simulink model "Square_Wave_Injection"  (R2023b)
settings: Solver=VariableStepAuto  StartTime=0.0  StopTime=3  RelTol=1e-3
undefined symbols (not defined in the file or in its folder): DiscIntNeverNeededParam
libraries: spsDCVoltageSourceLib x1, spsPermanentMagnetSynchronousMachineLib x1, simulink x1, spsUniversalBridgeLib x1, sps_lib x1
settings Model: Creator=yfp  LastModifiedBy=13571
settings SolverCC: AlgebraicLoopSolver=TrustRegion
settings OptimizationCC: ReuseModelBlockBuffer=off
settings DebuggingCC: UnconnectedInputMsg=warning  UnconnectedOutputMsg=warning  UnconnectedLineMsg=warning  ArithmeticOperatorsInVariantConditions=warning
settings ModelReferenceCC: EnableRefExpFcnMdlSchedulingChecks=on
settings SFSimCC: CustomCodeUndefinedFunction=UseInterfaceOnly

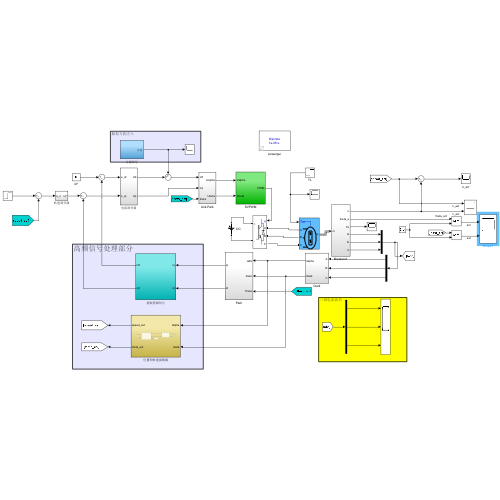
[thumbnail: Simulink's stored preview of the top-level diagram]
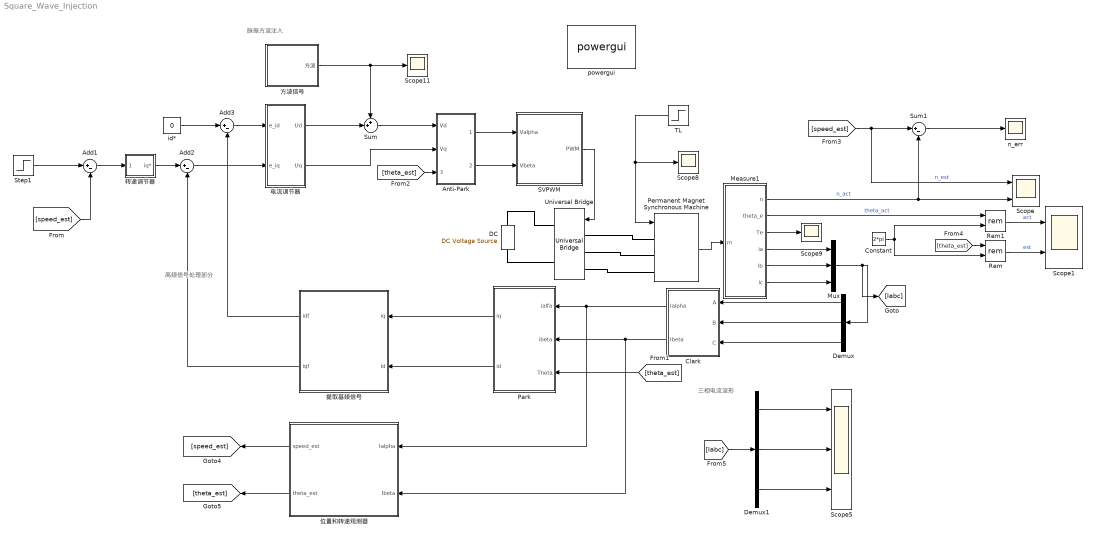
== system Square_Wave_Injection ==
  note: 三相电流波形
  note: 脉振方波注入
  note: 高频信号处理部分
  Add1 : Sum  Inputs=|+-
  Add2 : Sum  Inputs=|+-
  Add3 : Sum  Inputs=|+-
  Anti-Park : Subsystem
  Clark : Subsystem
  Constant : Constant  Value=2*pi
  "DC " : spsDCVoltageSourceLib/DC Voltage Source  Amplitude=300  Measurements=None
  Demux : Demux  Outputs=3
  Demux1 : Demux  Outputs=3
  Measure1 : Subsystem
  Mux : Mux  Inputs=3
  "Park " : Subsystem
  Permanent Magnet Synchronous Machine : spsPermanentMagnetSynchronousMachineLib/Permanent Magnet Synchronous Machine  NbPhases=3  FluxDistribution=Sinusoidal  RotorType=Salient-pole  MechanicalLoad=Torque Tm  PresetModel=No  ShowDetailedParameters=on  MeasurementBus=off  Resistance=0.045  Inductance=8.5e-3  dqInductances=[130e-6,235e-6]  La=0.000835  MachineConstant=Flux linkage established by magnets (V.s)  Flux=0.048517  VoltageCst=35.2  TorqueCst=0.2911  Flat=120  Mechanical=[0.0034 0.005 4 0]  PolePairs=4  InitialConditions=[0,0, 0,0]  InitialConditions5ph=[0 0 0 0 0 0]  RefAngle=Aligned with phase A axis (original Park)  IterativeDiscreteModel=Trapezoidal non iterative  TsBlock=-1  TsPowergui=0
  Rem : Math  Operator=rem  SignedPower=on
  Rem1 : Math  Operator=rem  SignedPower=on
  SVPWM : Subsystem
  Scope : Scope  NumInputPorts=2
  Scope1 : Scope  NumInputPorts=2
  Scope11 : Scope
  Scope5 : Scope  NumInputPorts=3
  Scope8 : Scope
  Scope9 : Scope
  Step1 : Step  Time=0  After=200  SampleTime=0
  Sum : Sum  Inputs=++|
  Sum1 : Sum  Inputs=|+-
  TL : Step  Time=0.5  SampleTime=0
  Universal Bridge : spsUniversalBridgeLib/Universal Bridge  Arms=3  SnubberResistance=1e5  SnubberCapacitance=inf  Device=IGBT / Diodes  Ron=1e-3  Lon=0  ForwardVoltages="[  0  0  ]"  ForwardVoltage=0  GTOparameters=[ 10e-6 , 20e-6 ]  IGBTparameters=[ 1e-6 , 2e-6 ]  Measurements=None  Measurements_2=None  converterType=Rectifier
  id* : Constant  Value=0
  n_err : Scope
  powergui : sps_lib/powergui  Priority=1  SimulationMode=Discrete  SampleTime=1e-6  frequency=60  Iterations=50  frequencyindice=0  Pbase=100e6  ErrMax=1e-4  UnitsV=kV  UnitsW=MW  buscounter=0  FunctionMessages=off  echomessages=off  EnableUseOfTLC=off  CurrentSourceSwitches=off  DisableSnubberDevices=off  DisableRonSwitches=off  DisableVfSwitches=off  DisplayEquations=off  AutomaticDiscreteSolvers=off  SolverType=Tustin/Backward Euler (TBE)  Interpol=off  ExternalGateDelay=off  methode=off  Ts=100  x0status=blocks  SPID=on  SwTol=0  HookPort=off  NonlinearTolerance=1e-4  nMaxIteration=100  ContinueOnMaxIteration=off  RestoreLinks=warning  ResistiveCurrentMeasurement=off  Frange=[0:2:500]  Ylog=off  Xlog=on  ShowGrid=off  save=off  variable=ZData  structure=iq  ZoomFFT=off  StartTime=0.1  cycles=100  DisplayStyle=2  fundamental=1000  FreqAxis=off  MaxFrequency=10000  frequencyindicesteady=1  RmsSteady=1  display=off
  位置和转速观测器 : Subsystem
  提取基频信号 : Subsystem
  方波信号 : Subsystem
  电流调节器 : Subsystem
  转速调节器 : Subsystem
  wires:
  Measure1/2(theta_e) -> Rem1/1  "theta_act"
  Sum/1 -> Anti-Park/1(Vd)
  Demux/2 -> Clark/2(B)
  Measure1/1(n) -> Sum1/2, Scope/2  "n_act"
  电流调节器/2(Uq) -> Anti-Park/2(Vq)
  电流调节器/1(Ud) -> Sum/2
  [speed_est] -> Scope/1, Sum1/1  "n_est"
  Step1/1 -> Add1/1
  Measure1/5(ib) -> Mux/2
  Sum1/1 -> n_err/1
  位置和转速观测器/2(theta_est) -> [theta_est]
  Add1/1 -> 转速调节器/1(e_n)
  Clark/2(Ibeta) -> 位置和转速观测器/2(Ibeta), "Park "/2(ibeta)
  位置和转速观测器/1(speed_est) -> [speed_est]
  Constant/1 -> Rem1/2, Rem/2
  Add2/1 -> 电流调节器/2(e_iq)
  "Park "/2(id) -> 提取基频信号/2(id)
  提取基频信号/1(idf) -> Add3/2
  Permanent Magnet Synchronous Machine/1 -> Measure1/1(m)
  Mux/1 -> [Iabc], Demux/1
  Demux/3 -> Clark/3(C)
  Measure1/3(Te) -> Scope9/1
  [theta_est] -> Rem/1
  TL/1 -> Scope8/1, Permanent Magnet Synchronous Machine/1
  Measure1/6(ic) -> Mux/3
  方波信号/1(方波) -> Scope11/1, Sum/1
  "Park "/1(iq) -> 提取基频信号/1(iq)
  Anti-Park/2(Ubeta) -> SVPWM/2(Vbeta)
  Measure1/4(ia) -> Mux/1
  Rem/1 -> Scope1/2  "est"
  Anti-Park/1(Ualpha) -> SVPWM/1(Valpha)
  Demux/1 -> Clark/1(A)
  Add3/1 -> 电流调节器/1(e_id)
  id*/1 -> Add3/1
  Rem1/1 -> Scope1/1  "act"
  提取基频信号/2(iqf) -> Add2/2
  Clark/1(Ialpha) -> 位置和转速观测器/1(Ialpha), "Park "/1(ialfa)
  [speed_est] -> Add1/2
  [theta_est] -> Anti-Park/3(theta)
  [theta_est] -> "Park "/3(Theta)
  SVPWM/1(PWM) -> Universal Bridge/1
  转速调节器/1(iq*) -> Add2/1
  [Iabc] -> Demux1/1
  Demux1/1 -> Scope5/1
  Demux1/2 -> Scope5/2
  Demux1/3 -> Scope5/3
  connections:
  Permanent Magnet Synchronous Machine/LConn1 -- Universal Bridge/LConn1
  Permanent Magnet Synchronous Machine/LConn3 -- Universal Bridge/LConn3
  "DC "/LConn1 -- Universal Bridge/RConn2
  Universal Bridge/RConn1 -- "DC "/RConn1
  Permanent Magnet Synchronous Machine/LConn2 -- Universal Bridge/LConn2

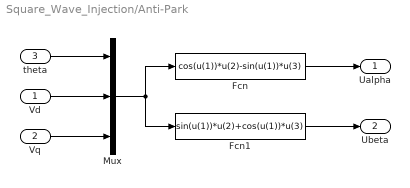
== system Square_Wave_Injection/Anti-Park ==
  Vd : Inport
  Vq : Inport  Port=2
  theta : Inport  Port=3
  Fcn : Fcn  Expr=cos(u(1))*u(2)-sin(u(1))*u(3)
  Fcn1 : Fcn  Expr=sin(u(1))*u(2)+cos(u(1))*u(3)
  Mux : Mux  Inputs=3
  Ualpha : Outport  VectorParamsAs1DForOutWhenUnconnected=off
  Ubeta : Outport  Port=2  VectorParamsAs1DForOutWhenUnconnected=off
  wires:
  Vd/1 -> Mux/2
  Vq/1 -> Mux/3
  Mux/1 -> Fcn/1, Fcn1/1
  Fcn1/1 -> Ubeta/1
  Fcn/1 -> Ualpha/1
  theta/1 -> Mux/1

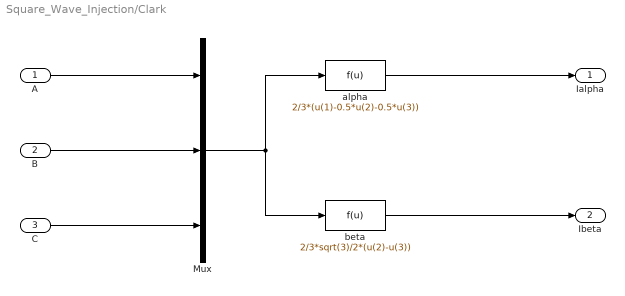
== system Square_Wave_Injection/Clark ==
  A : Inport
  B : Inport  Port=2
  C : Inport  Port=3
  Mux : Mux  Inputs=3
  alpha : Fcn  Expr=2/3*(u(1)-0.5*u(2)-0.5*u(3))
  beta : Fcn  Expr=2/3*sqrt(3)/2*(u(2)-u(3))
  Ialpha : Outport  VectorParamsAs1DForOutWhenUnconnected=off
  Ibeta : Outport  Port=2  VectorParamsAs1DForOutWhenUnconnected=off
  wires:
  Mux/1 -> beta/1, alpha/1
  alpha/1 -> Ialpha/1
  beta/1 -> Ibeta/1
  C/1 -> Mux/3
  A/1 -> Mux/1
  B/1 -> Mux/2

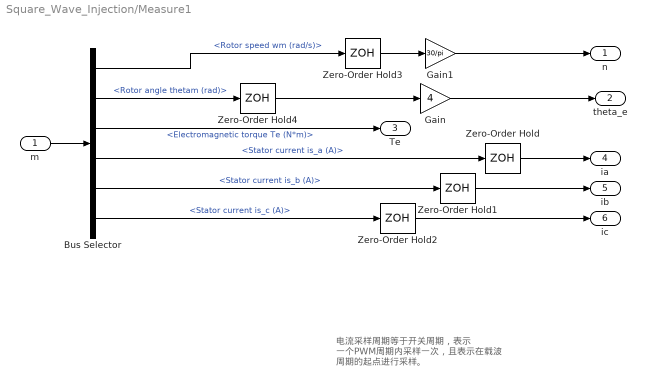
== system Square_Wave_Injection/Measure1 ==
  note: 电流采样周期等于开关周期，表示
      | 一个PWM周期内采样一次，且表示在载波
      | 周期的起点进行采样。
  m : Inport
  Bus Selector : BusSelector  OutputSignals=Rotor speed wm (rad/s),Rotor angle thetam (rad),Electromagnetic torque Te (N*m),Stator current is_a (A),Stator current is_b (A),Stator current is_c (A)
  Gain : Gain  Gain=4
  Gain1 : Gain  Gain=30/pi
  Zero-Order Hold{,1..4} (5 alike) : ZeroOrderHold  SampleTime=1e-4
  n : Outport  VectorParamsAs1DForOutWhenUnconnected=off
  theta_e : Outport  Port=2  VectorParamsAs1DForOutWhenUnconnected=off
  Te : Outport  Port=3  VectorParamsAs1DForOutWhenUnconnected=off
  ia : Outport  Port=4  VectorParamsAs1DForOutWhenUnconnected=off
  ib : Outport  Port=5  VectorParamsAs1DForOutWhenUnconnected=off
  ic : Outport  Port=6  VectorParamsAs1DForOutWhenUnconnected=off
  wires:
  m/1 -> Bus Selector/1
  Bus Selector/3 -> Te/1  "<Electromagnetic torque Te (N*m)>"
  Bus Selector/1 -> Zero-Order Hold3/1  "<Rotor speed wm (rad/s)>"
  Bus Selector/2 -> Zero-Order Hold4/1  "<Rotor angle thetam (rad)>"
  Bus Selector/4 -> Zero-Order Hold/1  "<Stator current is_a (A)>"
  Bus Selector/5 -> Zero-Order Hold1/1  "<Stator current is_b (A)>"
  Bus Selector/6 -> Zero-Order Hold2/1  "<Stator current is_c (A)>"
  Zero-Order Hold3/1 -> Gain1/1
  Zero-Order Hold4/1 -> Gain/1
  Zero-Order Hold/1 -> ia/1
  Zero-Order Hold1/1 -> ib/1
  Zero-Order Hold2/1 -> ic/1
  Gain/1 -> theta_e/1
  Gain1/1 -> n/1

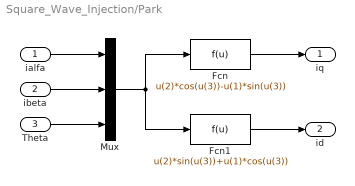
== system Square_Wave_Injection/Park  ==
  ialfa : Inport
  ibeta : Inport  Port=2
  Theta : Inport  Port=3
  Fcn : Fcn  Expr=u(2)*cos(u(3))-u(1)*sin(u(3))
  Fcn1 : Fcn  Expr=u(2)*sin(u(3))+u(1)*cos(u(3))
  Mux : Mux  Inputs=3
  iq : Outport  VectorParamsAs1DForOutWhenUnconnected=off
  id : Outport  Port=2  VectorParamsAs1DForOutWhenUnconnected=off
  wires:
  Theta/1 -> Mux/3
  Fcn1/1 -> id/1
  Fcn/1 -> iq/1
  Mux/1 -> Fcn/1, Fcn1/1
  ibeta/1 -> Mux/2
  ialfa/1 -> Mux/1

== system Square_Wave_Injection/SVPWM ==
  Valpha : Inport
  Vbeta : Inport  Port=2
  CMPR : Scope
  Embedded MATLAB Function : MATLAB Function  TreatAsAtomicUnit=on
  Mux6 : Mux  Inputs=3
  Udc : Constant  Value=135
  pwm generator : Subsystem
  PWM : Outport  VectorParamsAs1DForOutWhenUnconnected=off
  wires:
  Embedded MATLAB Function/1(ta) -> Mux6/1, pwm generator/1(Ta)
  Embedded MATLAB Function/2(tb) -> Mux6/2, pwm generator/2(Tb)
  Embedded MATLAB Function/3(tc) -> Mux6/3, pwm generator/3(Tc)
  Mux6/1 -> CMPR/1
  pwm generator/1(pwm) -> PWM/1
  Valpha/1 -> Embedded MATLAB Function/1(Vsalpha)
  Vbeta/1 -> Embedded MATLAB Function/2(Vsbeta)
  Udc/1 -> Embedded MATLAB Function/3(Udc)

== system Square_Wave_Injection/位置和转速观测器 ==
  Ialpha : Inport
  Ibeta : Inport  Port=2
  两相静止坐标系提取高频信号 : Subsystem
  位置估算2 : Subsystem
  speed_est : Outport
  theta_est : Outport  Port=2
  wires:
  Ialpha/1 -> 两相静止坐标系提取高频信号/1(i_alpha)
  Ibeta/1 -> 两相静止坐标系提取高频信号/2(i_beta)
  两相静止坐标系提取高频信号/1(i_alpha_h) -> 位置估算2/1(Ialpha_h)
  两相静止坐标系提取高频信号/2(i_beta_h) -> 位置估算2/2(Ibeta_h)
  [Udh] -> 位置估算2/3(Udh)
  位置估算2/1(Speed_Est) -> speed_est/1
  位置估算2/2(theta_e^) -> theta_est/1

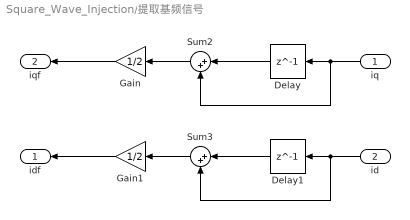
== system Square_Wave_Injection/提取基频信号 ==
  iq : Inport
  id : Inport  Port=2
  Delay : Delay  DelayLength=1  SampleTime=1e-4
  Delay1 : Delay  DelayLength=1  SampleTime=1e-4
  Gain : Gain  Gain=1/2
  Gain1 : Gain  Gain=1/2
  Sum2 : Sum  Inputs=|++
  Sum3 : Sum  Inputs=|++
  idf : Outport  VectorParamsAs1DForOutWhenUnconnected=off
  iqf : Outport  Port=2  VectorParamsAs1DForOutWhenUnconnected=off
  wires:
  Delay/1 -> Sum2/1
  Delay1/1 -> Sum3/1
  Sum3/1 -> Gain1/1
  id/1 -> Delay1/1, Sum3/2
  Gain1/1 -> idf/1
  Gain/1 -> iqf/1
  Sum2/1 -> Gain/1
  iq/1 -> Delay/1, Sum2/2

== system Square_Wave_Injection/方波信号 ==
  Constant : Constant  Value=20
  Pulse Generator : DiscretePulseGenerator  PulseType=Time based  Amplitude=40  Period=2e-4  PulseWidth=50
  Subtract : Sum  Inputs=+-
  方波 : Outport  VectorParamsAs1DForOutWhenUnconnected=off
  tag scope: Udh=global
  wires:
  Pulse Generator/1 -> Subtract/1
  Constant/1 -> Subtract/2
  Subtract/1 -> [Udh], 方波/1

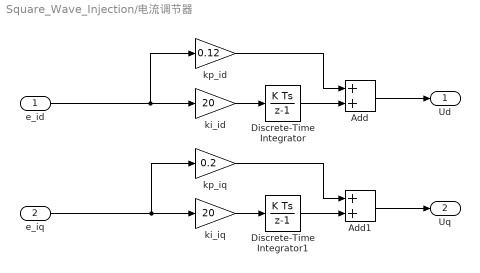
== system Square_Wave_Injection/电流调节器 ==
  e_id : Inport
  e_iq : Inport  Port=2
  Add : Sum
  Add1 : Sum
  Discrete-Time Integrator : DiscreteIntegrator  SampleTime=1e-4  LimitOutput=on  UpperSaturationLimit=135/1.732  LowerSaturationLimit=-135/1.732  ICPrevOutput=DiscIntNeverNeededParam  ICPrevScaledInput=DiscIntNeverNeededParam
  Discrete-Time Integrator1 : DiscreteIntegrator  SampleTime=1e-4  LimitOutput=on  UpperSaturationLimit=135/1.732  LowerSaturationLimit=-135/1.732  ICPrevOutput=DiscIntNeverNeededParam  ICPrevScaledInput=DiscIntNeverNeededParam
  ki_id : Gain  Gain=20
  ki_iq : Gain  Gain=20
  kp_id : Gain  Gain=0.12
  kp_iq : Gain  Gain=0.2
  Ud : Outport  VectorParamsAs1DForOutWhenUnconnected=off
  Uq : Outport  Port=2  VectorParamsAs1DForOutWhenUnconnected=off
  wires:
  ki_id/1 -> Discrete-Time Integrator/1
  Discrete-Time Integrator/1 -> Add/2
  kp_id/1 -> Add/1
  ki_iq/1 -> Discrete-Time Integrator1/1
  Discrete-Time Integrator1/1 -> Add1/2
  kp_iq/1 -> Add1/1
  Add/1 -> Ud/1
  Add1/1 -> Uq/1
  e_id/1 -> kp_id/1, ki_id/1
  e_iq/1 -> kp_iq/1, ki_iq/1

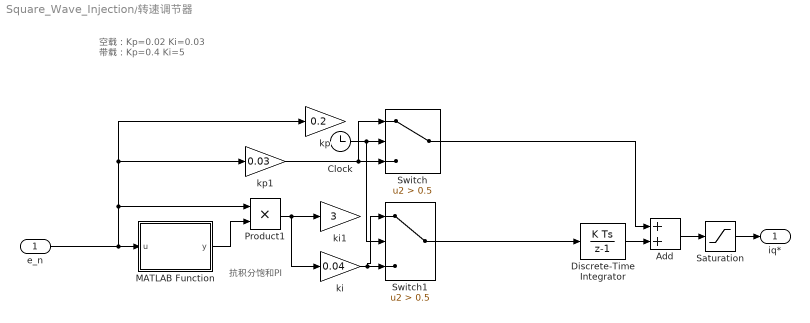
== system Square_Wave_Injection/转速调节器 ==
  note: 空载：Kp=0.02 Ki=0.03
      | 带载：Kp=0.4 Ki=5
  note: 抗积分饱和PI
  e_n : Inport
  Add : Sum
  Clock : Clock
  Discrete-Time Integrator : DiscreteIntegrator  SampleTime=1e-4  LimitOutput=on  UpperSaturationLimit=50  LowerSaturationLimit=-50  ICPrevOutput=DiscIntNeverNeededParam  ICPrevScaledInput=DiscIntNeverNeededParam
  MATLAB Function : MATLAB Function  TreatAsAtomicUnit=on
  Product1 : Product
  Saturation : Saturate  UpperLimit=50  LowerLimit=-50
  Switch : Switch  Criteria=u2 > Threshold  Threshold=0.5  SaturateOnIntegerOverflow=off  InputSameDT=off
  Switch1 : Switch  Criteria=u2 > Threshold  Threshold=0.5  SaturateOnIntegerOverflow=off  InputSameDT=off
  ki : Gain  Gain=0.04
  ki1 : Gain  Gain=3
  kp : Gain  Gain=0.2
  kp1 : Gain  Gain=0.03
  iq* : Outport  VectorParamsAs1DForOutWhenUnconnected=off
  wires:
  Discrete-Time Integrator/1 -> Add/2
  Add/1 -> Saturation/1
  MATLAB Function/1(y) -> Product1/2
  Saturation/1 -> iq*/1
  e_n/1 -> kp/1, kp1/1, Product1/1, MATLAB Function/1(u)
  Clock/1 -> Switch1/2, Switch/2
  Product1/1 -> ki/1, ki1/1
  Switch/1 -> Add/1
  Switch1/1 -> Discrete-Time Integrator/1
  ki/1 -> Switch1/1, Switch1/3
  kp1/1 -> Switch/1, Switch/3

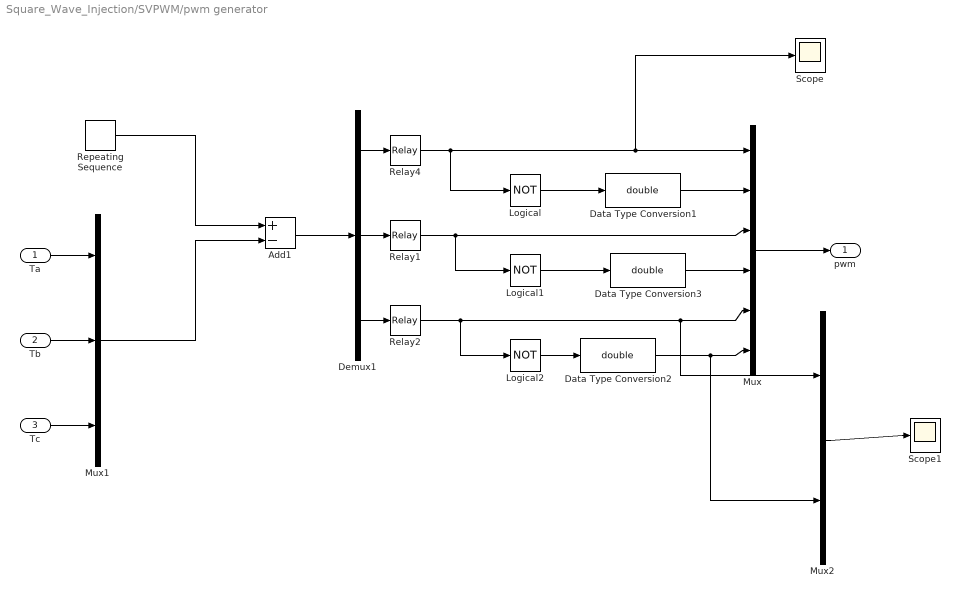
== system Square_Wave_Injection/SVPWM/pwm generator ==
  Ta : Inport
  Tb : Inport  Port=2
  Tc : Inport  Port=3
  Add1 : Sum  Inputs=+-
  Data Type Conversion1 : DataTypeConversion  OutDataTypeStr=double  SaturateOnIntegerOverflow=off  RndMeth=Floor
  Data Type Conversion2 : DataTypeConversion  OutDataTypeStr=double  SaturateOnIntegerOverflow=off  RndMeth=Floor
  Data Type Conversion3 : DataTypeConversion  OutDataTypeStr=double  SaturateOnIntegerOverflow=off  RndMeth=Floor
  Demux1 : Demux  Outputs=3
  "Logical " : Logic  Operator=NOT  AllPortsSameDT=off  OutDataTypeStr=boolean
  Logical1 : Logic  Operator=NOT  AllPortsSameDT=off  OutDataTypeStr=boolean
  Logical2 : Logic  Operator=NOT  AllPortsSameDT=off  OutDataTypeStr=boolean
  Mux : Mux  Inputs=6
  Mux1 : Mux  Inputs=3
  Mux2 : Mux  Inputs=2
  Relay1 : Relay  OnSwitchValue=0.00001  OffSwitchValue=-0.00001  OutDataTypeStr=Inherit: Inherit via back propagation
  Relay2 : Relay  OnSwitchValue=0.00001  OffSwitchValue=-0.00001  OutDataTypeStr=Inherit: Inherit via back propagation
  Relay4 : Relay  OnSwitchValue=0.00001  OffSwitchValue=-0.00001  OutDataTypeStr=Inherit: Inherit via back propagation
  Repeating Sequence : simulink/Sources/Repeating Sequence  rep_seq_t=[0 0.00005 0.0001]  rep_seq_y=[0 1 0]
  Scope : Scope
  Scope1 : Scope
  pwm : Outport  VectorParamsAs1DForOutWhenUnconnected=off
  wires:
  Repeating Sequence/1 -> Add1/1
  Demux1/1 -> Relay4/1
  Demux1/2 -> Relay1/1
  Demux1/3 -> Relay2/1
  Mux/1 -> pwm/1
  Add1/1 -> Demux1/1
  "Logical "/1 -> Data Type Conversion1/1
  Data Type Conversion1/1 -> Mux/2
  Logical1/1 -> Data Type Conversion3/1
  Data Type Conversion3/1 -> Mux/4
  Logical2/1 -> Data Type Conversion2/1
  Data Type Conversion2/1 -> Mux/6, Mux2/2
  Relay4/1 -> "Logical "/1, Mux/1, Scope/1
  Relay1/1 -> Logical1/1, Mux/3
  Relay2/1 -> Logical2/1, Mux/5, Mux2/1
  Ta/1 -> Mux1/1
  Tb/1 -> Mux1/2
  Tc/1 -> Mux1/3
  Mux1/1 -> Add1/2
  Mux2/1 -> Scope1/1

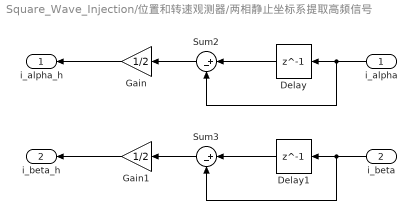
== system Square_Wave_Injection/位置和转速观测器/两相静止坐标系提取高频信号 ==
  i_alpha : Inport
  i_beta : Inport  Port=2
  Delay : Delay  DelayLength=1  SampleTime=1e-4
  Delay1 : Delay  DelayLength=1  SampleTime=1e-4
  Gain : Gain  Gain=1/2
  Gain1 : Gain  Gain=1/2
  Sum2 : Sum  Inputs=|+-
  Sum3 : Sum  Inputs=|+-
  i_alpha_h : Outport  VectorParamsAs1DForOutWhenUnconnected=off
  i_beta_h : Outport  Port=2  VectorParamsAs1DForOutWhenUnconnected=off
  wires:
  i_alpha/1 -> Sum2/2, Delay/1
  Sum2/1 -> Gain/1
  Gain/1 -> i_alpha_h/1
  Gain1/1 -> i_beta_h/1
  i_beta/1 -> Sum3/2, Delay1/1
  Sum3/1 -> Gain1/1
  Delay1/1 -> Sum3/1
  Delay/1 -> Sum2/1

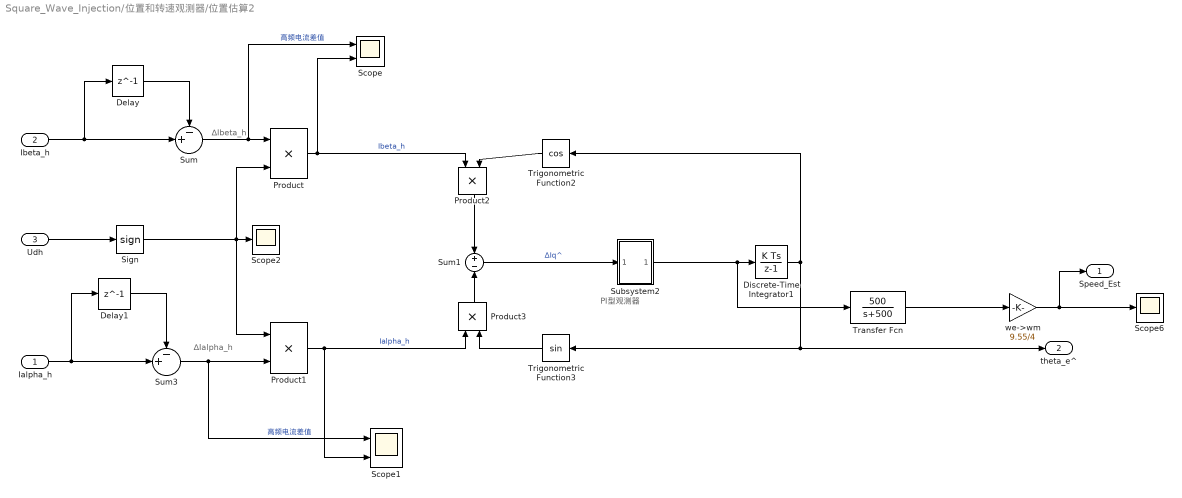
== system Square_Wave_Injection/位置和转速观测器/位置估算2 ==
  note: PI型观测器
  note: ∆Ialpha_h
  note: ∆Ibeta_h
  Ialpha_h : Inport
  Ibeta_h : Inport  Port=2
  Udh : Inport  Port=3
  Delay : Delay  DelayLength=1  SampleTime=1e-4
  Delay1 : Delay  DelayLength=1  SampleTime=1e-4
  Discrete-Time Integrator1 : DiscreteIntegrator  SampleTime=1e-4  ICPrevOutput=DiscIntNeverNeededParam  ICPrevScaledInput=DiscIntNeverNeededParam
  Product{,1..3} (4 alike) : Product
  Scope : Scope  NumInputPorts=2
  Scope1 : Scope  NumInputPorts=2
  Scope2 : Scope
  Scope6 : Scope
  Sign : Signum
  Subsystem2 : Subsystem  mask{Kp=10, Ki=25, UpperLimit=2*pi*6000/15, LowerLimit=-2*pi*6000/15}
      mask Display: disp('PI')
  Sum : Sum  Inputs=-+|
  Sum1 : Sum  Inputs=+|-
  Sum3 : Sum  Inputs=-+|
  Transfer Fcn : TransferFcn  Numerator=[500]  Denominator=[1 500]
  Trigonometric Function2 : Trigonometry  Operator=cos
  Trigonometric Function3 : Trigonometry
  we->wm : Gain  Gain=9.55/4
  Speed_Est : Outport  VectorParamsAs1DForOutWhenUnconnected=off
  theta_e^ : Outport  Port=2  VectorParamsAs1DForOutWhenUnconnected=off
  wires:
  Transfer Fcn/1 -> we->wm/1
  Discrete-Time Integrator1/1 -> theta_e^/1, Trigonometric Function3/1, Trigonometric Function2/1
  Trigonometric Function2/1 -> Product2/2
  Product2/1 -> Sum1/1
  Trigonometric Function3/1 -> Product3/2
  Sum1/1 -> Subsystem2/1(In1)  "∆Iq^"
  Product3/1 -> Sum1/2
  Subsystem2/1(Out1) -> Discrete-Time Integrator1/1, Transfer Fcn/1
  we->wm/1 -> Scope6/1, Speed_Est/1
  Ialpha_h/1 -> Sum3/2, Delay1/1
  Ibeta_h/1 -> Delay/1, Sum/2
  Delay/1 -> Sum/1
  Delay1/1 -> Sum3/1
  Product/1 -> Scope/2, Product2/1  "Ibeta_h"
  Sum/1 -> Scope/1, Product/1  "高频电流差值"
  Sum3/1 -> Scope1/1, Product1/2  "高频电流差值"
  Product1/1 -> Scope1/2, Product3/1  "Ialpha_h"
  Sign/1 -> Scope2/1, Product/2, Product1/1
  Udh/1 -> Sign/1

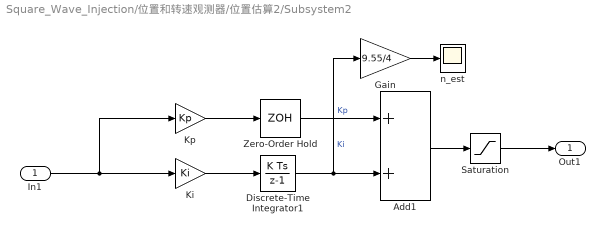
== system Square_Wave_Injection/位置和转速观测器/位置估算2/Subsystem2 ==
  In1 : Inport
  Add1 : Sum
  Discrete-Time Integrator1 : DiscreteIntegrator  SampleTime=1e-4  LimitOutput=on  UpperSaturationLimit=UpperLimit  LowerSaturationLimit=LowerLimit  ICPrevOutput=DiscIntNeverNeededParam  ICPrevScaledInput=DiscIntNeverNeededParam
  Gain : Gain  Gain=9.55/4
  Ki : Gain  Gain=Ki
  Kp : Gain  Gain=Kp
  Saturation : Saturate  UpperLimit=UpperLimit  LowerLimit=LowerLimit
  Zero-Order Hold : ZeroOrderHold  SampleTime=1e-4
  n_est : Scope
  Out1 : Outport  VectorParamsAs1DForOutWhenUnconnected=off
  wires:
  In1/1 -> Kp/1, Ki/1
  Ki/1 -> Discrete-Time Integrator1/1
  Zero-Order Hold/1 -> Add1/1  "Kp"
  Add1/1 -> Saturation/1
  Discrete-Time Integrator1/1 -> Gain/1, Add1/2  "Ki"
  Saturation/1 -> Out1/1
  Kp/1 -> Zero-Order Hold/1
  Gain/1 -> n_est/1

== matlab function Square_Wave_Injection/SVPWM/Embedded MATLAB Function ==
  data: Vsalpha input; Vsbeta input; ta output; tb output; tc output; Udc input
function [ta,tb,tc]= f(Vsalpha,Vsbeta,Udc)
ta=0;tb=0;tc=0;Ts=2;

va=Vsbeta;
vb=-(Vsalpha*sqrt(3)+Vsbeta)/2;
vc=(Vsalpha*sqrt(3)-Vsbeta)/2;

a=0;b=0;c=0;sector=0;
if va>0
    a=1;
end
if vb>0
    b=1;
end
if vc>0
    c=1;
end
sector=a+2*b+4*c;

x=sqrt(3)*Vsbeta*Ts/Udc;
y=(3*Vsalpha+sqrt(3)*Vsbeta)*Ts/(2*Udc);
z=(-3*Vsalpha+sqrt(3)*Vsbeta)*Ts/(2*Udc);

t1=0;t2=0;

switch sector
    case 1
        t1=z;
        t2=y;
    case 2
        t1=-x;
        t2=z;
    case 3
        t1=x;
        t2=-y;
    case 4
        t1=y;
        t2=-x;
    case 5
        t1=-z;
        t2=x;
    case 6
        t1=-y;
        t2=-z;
end

t11=t1; t12=t2;
if (t1+t2)>Ts
    t1=t11/(t11+t12)*Ts;
    t2=t12/(t11+t12)*Ts;
end
t0=Ts-t1-t2;

tcm1=t0/4;
tcm2=tcm1+t1/2;
tcm3=tcm2+t2/2;

switch sector
    case 1
        ta=tcm2;
        tb=tcm1;
        tc=tcm3;
    case 2
        ta=tcm3;
        tb=tcm2;
        tc=tcm1;
    case 3
        ta=tcm3;
        tb=tcm1;
        tc=tcm2;
    case 4
        ta=tcm1;
        tb=tcm3;
        tc=tcm2;
    case 5
        ta=tcm1;
        tb=tcm2;
        tc=tcm3;
    case 6
        ta=tcm2;
        tb=tcm3;
        tc=tcm1;
end

== matlab function Square_Wave_Injection/转速调节器/MATLAB Function ==
  data: u input; y output
function y = fcn(u)
if (abs(u)>300)
    y=0;
else
    y=1;
end
